simulink model "ChiefMaster_TTC580"  (R2022b)
settings: Solver=FixedStepAuto  StartTime=0.0  StopTime=10  FixedStep=0.01  RelTol=1e-3
values from neighbouring files (symbols this model uses):
  BattBox1_No = single(1)    [Parameters.m]
  BattBox2_No = single(2)    [Parameters.m]
  BattBox3_No = single(3)    [Parameters.m]
  CurrentLB = single(-3)    [Parameters.m]
  CurrentReductionConstant_Lvl0 = single(0.03)    [Parameters.m]
  CurrentReductionConstant_Lvl1 = single(0.05)    [Parameters.m]
  CurrentReductionConstant_Lvl2 = single(0.07)    [Parameters.m]
  CurrentReductionConstant_Lvl3 = single(0.1)    [Parameters.m]
  CurrentUB = single(3)    [Parameters.m]
  DCHV_Minus_In_Delay_ms = single(500)    [Parameters.m]
  FL_sHVC_CellBalanceVoltage_mV = single(3500)    [Parameters.m]
  FL_sInrushCurrent_dividebyzero = single(0.00001)    [Parameters.m]
  FL_u8HMI_BuzzerTimer = uint8(3)    [Parameters.m]
  IP_boActValue = true    [Parameters.m]
  IP_boDeactValue = false    [Parameters.m]
  IP_boInitValue = false    [Parameters.m]
  IP_s_LB = 18000    [Parameters.m]
  IP_s_UB = 22000    [Parameters.m]
  IP_sBatt1_ChargeCurrentMax_Factor = single(0.1)    [Parameters.m]
  IP_sBatt1_ChargeCurrentMax_LB = single(0)    [Parameters.m]
  IP_sBatt1_ChargeCurrentMax_Offset = single(0)    [Parameters.m]
  IP_sBatt1_ChargeCurrentMax_UB = single(6553.5)    [Parameters.m]
  IP_sBatt1_Current_Factor = single(0.1)    [Parameters.m]
  IP_sBatt1_Current_LB = single(-3276.8)    [Parameters.m]
  IP_sBatt1_Current_Offset = single(0)    [Parameters.m]
  IP_sBatt1_Current_UB = single(3276.8)    [Parameters.m]
  IP_sBatt1_DisChargeCurrentMax_Factor = single(0.1)    [Parameters.m]
  IP_sBatt1_DisChargeCurrentMax_LB = single(0)    [Parameters.m]
  IP_sBatt1_DisChargeCurrentMax_Offset = single(0)    [Parameters.m]
  IP_sBatt1_DisChargeCurrentMax_UB = single(6553.5)    [Parameters.m]
  IP_sBatt1_InsulationResistance_Factor = single(5)    [Parameters.m]
  IP_sBatt1_InsulationResistance_LB = single(0)    [Parameters.m]
  IP_sBatt1_InsulationResistance_Offset = single(0)    [Parameters.m]
  IP_sBatt1_InsulationResistance_UB = single(0)    [Parameters.m]
  IP_sBatt1_LiBa_IntResist_mOhm = single(25)    [Parameters.m]
  IP_sBatt1_SOC_Factor = single(1)    [Parameters.m]
  IP_sBatt1_SOC_LB = single(0)    [Parameters.m]
  IP_sBatt1_SOC_Offset = single(0)    [Parameters.m]
  IP_sBatt1_SOC_UB = single(100)    [Parameters.m]
  IP_sBatt1_SOH_Factor = single(1)    [Parameters.m]
  IP_sBatt1_SOH_LB = single(0)    [Parameters.m]
  IP_sBatt1_SOH_Offset = single(0)    [Parameters.m]
  IP_sBatt1_SOH_UB = single(100)    [Parameters.m]
  IP_sBatt1_Ubatt_Factor = single(0.1)    [Parameters.m]
  IP_sBatt1_Ubatt_LB = single(0)    [Parameters.m]
  IP_sBatt1_Ubatt_Offset = single(0)    [Parameters.m]
  IP_sBatt1_Ubatt_UB = single(6553.5)    [Parameters.m]
  IP_sBatt1_UserRi_Factor = single(1)    [Parameters.m]
  IP_sBatt1_UserRi_LB = single(0)    [Parameters.m]
  IP_sBatt1_UserRi_Offset = single(0)    [Parameters.m]
  IP_sBatt1_UserRi_UB = single(255)    [Parameters.m]
  IP_sBatt1_VoltageAtSensor_Factor = single(0.02)    [Parameters.m]
  IP_sBatt1_VoltageAtSensor_LB = single(0)    [Parameters.m]
  IP_sBatt1_VoltageAtSensor_Offset = single(0)    [Parameters.m]
  IP_sBatt1_VoltageAtSensor_UB = single(1310.7)    [Parameters.m]
  IP_sBatt2_LiBa_IntResist_mOhm = single(25)    [Parameters.m]
  IP_sBatt3_LiBa_IntResist_mOhm = single(25)    [Parameters.m]
  IP_sEM_LB = 2000    [Parameters.m]
  IP_sEM_UB = 8000    [Parameters.m]
  IP_sFB_LB = 5000    [Parameters.m]
  IP_sFB_UB = 10000    [Parameters.m]
  IP_sHVIL_LB = 12000    [Parameters.m]
  IP_sHVIL_UB = 15000    [Parameters.m]
  IP_sLoad_Voltage_Factor = single(1)    [Parameters.m]
  IP_sLoad_Voltage_LB = single(0)    [Parameters.m]
  IP_sLoad_Voltage_Offset = single(0)    [Parameters.m]
  IP_sLoad_Voltage_UB = single(65535)    [Parameters.m]
  IP_u8HVIL_Delay_ms = uint8(100)    [Parameters.m]
  IP_u8HW_IN_delay_ms = uint8(100)    [Parameters.m]
  IT_sInsulationSafeValue_kOhm = single(650)    [Parameters.m]
  IT_u8IMD_DelayTime_s = uint8(20)    [Parameters.m]
  MainHV_Minus_In_Delay = single(5)    [Parameters.m]
  MainHV_StatusDelay = single(5)    [Parameters.m]
  NotAvailable_uint16 = single(65535)    [Parameters.m]
  NotAvailable_uint8 = uint8(255)    [Parameters.m]
  OP_boHVIL_Supply = boolean(1)    [Parameters.m]
  SafeCurrentToCloseHV_A = single(5)    [Parameters.m]
  SafeVoltageToCloseHV_V = single(0.5)    [Parameters.m]
  UnexpectedBattChargingFcn_Available = boolean(1)    [Parameters.m]
  Voltage_NA_UB = uint16(65535)    [Parameters.m]
  VoltageSensorAvailableBB1 = boolean(0)    [Parameters.m]
  VoltageSensorAvailableBB2 = boolean(0)    [Parameters.m]
  VoltageSensorAvailableBB3 = boolean(0)    [Parameters.m]
libraries: simulink x184, Library_DataProcessing_v1_1 x167, Library_DataProcessing_v1 x142, libCM x28
(part 11 of 19)

== system ChiefMaster_TTC580/ChiefMaster/Input Processing/LiBa/LiBa_Box1/Subsystem13 ==
  C_LB_Batt1_CellVoltage01_Timeout : Inport
  C_LB_Batt1_CellVoltage02_Timeout : Inport  Port=2
  C_LB_Batt1_CellTemperature_Timeout : Inport  Port=3
  C_LB_Batt1_InsulationMonitor_Timeout : Inport  Port=4
  C_LB_Batt1_Status01_Timeout : Inport  Port=5
  C_LB_Batt1_Status02_Timeout : Inport  Port=6
  C_LB_Batt1_Status03_Timeout : Inport  Port=7
  AND : Logic  Inputs=7  AllPortsSameDT=off  OutDataTypeStr=boolean
  Constant : Constant  OutDataTypeStr=boolean
  Constant1 : Constant  Value=0  OutDataTypeStr=boolean
  NOT{,1..6} (7 alike) : Logic  Operator=NOT  AllPortsSameDT=off  OutDataTypeStr=boolean
  Switch : Switch  Criteria=u2 > Threshold  SaturateOnIntegerOverflow=off  InputSameDT=off
  IP_boLiBa_Batt1_Availability : Outport
  wires:
  NOT6/1 -> AND/7
  NOT5/1 -> AND/6
  C_LB_Batt1_Status03_Timeout/1 -> NOT6/1
  C_LB_Batt1_Status02_Timeout/1 -> NOT5/1
  C_LB_Batt1_Status01_Timeout/1 -> NOT4/1
  Switch/1 -> IP_boLiBa_Batt1_Availability/1  "IP_boLiBa_Batt1_Availability"
  C_LB_Batt1_CellVoltage01_Timeout/1 -> NOT/1
  C_LB_Batt1_CellVoltage02_Timeout/1 -> NOT1/1
  C_LB_Batt1_CellTemperature_Timeout/1 -> NOT2/1
  C_LB_Batt1_InsulationMonitor_Timeout/1 -> NOT3/1
  NOT/1 -> AND/1
  NOT1/1 -> AND/2
  NOT2/1 -> AND/3
  NOT3/1 -> AND/4
  NOT4/1 -> AND/5
  AND/1 -> Switch/2
  Constant/1 -> Switch/1
  Constant1/1 -> Switch/3

== system ChiefMaster_TTC580/ChiefMaster/Input Processing/LiBa/LiBa_Box2/BMS_CellTemperature ==
  C_LB_Batt2_CellTemperature_Msg : Inport
  C_LB_Batt2_CellTemperature_Timeout : Inport  Port=2
  Bus Creator1 : BusCreator  Inputs=7
  Demux : Demux  Outputs=8
  Subsystem : Subsystem
  Subsystem1 : Subsystem
  Subsystem2 : Subsystem
  Subsystem3 : Subsystem
  Subsystem4 : Subsystem
  Subsystem5 : Subsystem
  Subsystem6 : Subsystem
  Terminator1 : Terminator
  IP_LB_Batt2_CellTemperature_DataBus : Outport
  wires:
  Subsystem3/1(IP_LB_BMS_ACT_Cel_T_Min_Cel_DataBus) -> Bus Creator1/4
  [C_LB_BMS_CellTemperature_Timeout] -> Subsystem3/2(C_LB_BMS_CellTemperature_Timeout)
  Demux/4 -> Subsystem3/1(byte3)
  Demux/3 -> Subsystem2/1(byte2)
  Demux/2 -> Subsystem1/1(byte1)
  C_LB_Batt2_CellTemperature_Msg/1 -> Demux/1
  Demux/1 -> Subsystem/1(byte0)
  C_LB_Batt2_CellTemperature_Timeout/1 -> [C_LB_BMS_CellTemperature_Timeout]
  [C_LB_BMS_CellTemperature_Timeout] -> Subsystem/2(C_LB_BMS_CellTemperature_Timeout)
  [C_LB_BMS_CellTemperature_Timeout] -> Subsystem1/2(C_LB_BMS_CellTemperature_Timeout)
  [C_LB_BMS_CellTemperature_Timeout] -> Subsystem2/2(C_LB_BMS_CellTemperature_Timeout)
  Demux/8 -> Terminator1/1
  Subsystem/1(IP_LB_BMS_ACT_Cel_T_Avg_DataBus) -> Bus Creator1/1
  Subsystem1/1(IP_LB_BMS_ACT_Cel_T_Min_Value_DataBus) -> Bus Creator1/2
  Subsystem2/1(IP_LB_BMS_ACT_Cel_T_Max_Value_DataBus) -> Bus Creator1/3
  Bus Creator1/1 -> IP_LB_Batt2_CellTemperature_DataBus/1  "IP_LB_Batt2_CellTemperature_DataBus"
  [C_LB_BMS_CellTemperature_Timeout] -> Subsystem4/2(C_LB_BMS_CellTemperature_Timeout)
  [C_LB_BMS_CellTemperature_Timeout] -> Subsystem5/2(C_LB_BMS_CellTemperature_Timeout)
  [C_LB_BMS_CellTemperature_Timeout] -> Subsystem6/2(C_LB_BMS_CellTemperature_Timeout)
  Demux/5 -> Subsystem4/1(byte1)
  Demux/6 -> Subsystem5/1(byte2)
  Demux/7 -> Subsystem6/1(byte3)
  Subsystem4/1(IP_LB_BMS_ACT_Cel_T_Min_CMU_DataBus) -> Bus Creator1/5
  Subsystem5/1(IP_LB_BMS_ACT_Cel_T_Max_Cel_DataBus) -> Bus Creator1/6
  Subsystem6/1(IP_LB_BMS_ACT_Cel_V_Max_Cel_DataBus) -> Bus Creator1/7

== system ChiefMaster_TTC580/ChiefMaster/Input Processing/LiBa/LiBa_Box2/BMS_CellVoltage01 ==
  C_LB_Batt2_CellVoltage01_Msg : Inport
  C_LB_Batt2_CellVoltage01_Timeout : Inport  Port=2
  Bus Creator1 : BusCreator  Inputs=3
  Demux : Demux  Outputs=8
  Subsystem : Subsystem
  Subsystem1 : Subsystem
  Subsystem2 : Subsystem
  Terminator : Terminator
  Terminator1 : Terminator
  IP_LB_Batt2_CellVoltage01_DataBus : Outport
  wires:
  C_LB_Batt2_CellVoltage01_Msg/1 -> Demux/1
  Demux/1 -> Subsystem/1(byte0)
  Demux/2 -> Subsystem/2(byte1)
  C_LB_Batt2_CellVoltage01_Timeout/1 -> [C_LB_BMS_CellVoltage01_Timeout]
  [C_LB_BMS_CellVoltage01_Timeout] -> Subsystem/3(C_LB_CellVoltage01_Timeout)
  Demux/3 -> Subsystem1/1(byte2)
  Demux/4 -> Subsystem1/2(byte3)
  [C_LB_BMS_CellVoltage01_Timeout] -> Subsystem1/3(C_LB_CellVoltage01_Timeout)
  Demux/5 -> Subsystem2/1(byte4)
  Demux/6 -> Subsystem2/2(byte5)
  [C_LB_BMS_CellVoltage01_Timeout] -> Subsystem2/3(C_LB_CellVoltage01_Timeout)
  Demux/7 -> Terminator/1
  Demux/8 -> Terminator1/1
  Subsystem/1(IP_LB_BMS_ACT_Cel_mV_Min_DataBus) -> Bus Creator1/1
  Subsystem1/1(IP_LB_BMS_ACT_Cel_mV_AVG_DataBus) -> Bus Creator1/2
  Subsystem2/1(IP_LB_BMS_ACT_Cel_mV_Max_DataBus) -> Bus Creator1/3
  Bus Creator1/1 -> IP_LB_Batt2_CellVoltage01_DataBus/1  "IP_LB_Batt2_CellVoltage01_DataBus"

== system ChiefMaster_TTC580/ChiefMaster/Input Processing/LiBa/LiBa_Box2/BMS_CellVoltageNumber ==
  C_LB_Batt2_CellVoltage02_Msg : Inport
  C_LB_Batt2_CellVoltage02_Timeout : Inport  Port=2
  Bus Creator1 : BusCreator  Inputs=4
  Demux : Demux  Outputs=8
  Subsystem : Subsystem
  Subsystem1 : Subsystem
  Subsystem2 : Subsystem
  Subsystem3 : Subsystem
  Terminator{,1..3} (4 alike) : Terminator
  IP_LB_Batt2_CellVoltage02_DataBus : Outport
  wires:
  Bus Creator1/1 -> IP_LB_Batt2_CellVoltage02_DataBus/1  "IP_LB_Batt2_CellVoltage02_DataBus"
  Subsystem2/1(IP_LB_BMS_ACT_Cel_V_Max_Cel_DataBus) -> Bus Creator1/3
  Subsystem1/1(IP_LB_BMS_ACT_Cel_V_Min_CMU_DataBus) -> Bus Creator1/2
  Subsystem/1(IP_LB_BMS_ACT_Cel_V_Min_Cel_DataBus) -> Bus Creator1/1
  Demux/8 -> Terminator1/1
  Demux/7 -> Terminator/1
  [C_LB_BMS_CellVoltage02_Timeout] -> Subsystem2/2(C_LB_CellVoltage02_Timeout)
  [C_LB_BMS_CellVoltage02_Timeout] -> Subsystem1/2(C_LB_CellVoltage02_Timeout)
  [C_LB_BMS_CellVoltage02_Timeout] -> Subsystem/2(C_LB_CellVoltage02_Timeout)
  C_LB_Batt2_CellVoltage02_Timeout/1 -> [C_LB_BMS_CellVoltage02_Timeout]
  Demux/1 -> Subsystem/1(byte0)
  C_LB_Batt2_CellVoltage02_Msg/1 -> Demux/1
  Demux/2 -> Subsystem1/1(byte1)
  Demux/3 -> Subsystem2/1(byte2)
  Demux/4 -> Subsystem3/1(byte3)
  [C_LB_BMS_CellVoltage02_Timeout] -> Subsystem3/2(C_LB_CellVoltage02_Timeout)
  Subsystem3/1(IP_LB_BMS_ACT_Cel_V_Max_CMU_DataBus) -> Bus Creator1/4
  Demux/6 -> Terminator2/1
  Demux/5 -> Terminator3/1

== system ChiefMaster_TTC580/ChiefMaster/Input Processing/LiBa/LiBa_Box2/BMS_InsulationMonitor ==
  C_LB_Batt2_InsulationMonitor_Msg : Inport
  C_LB_Batt2_InsulationMonitor_Timeout : Inport  Port=2
  Bus Creator1 : BusCreator  Inputs=3
  Demux : Demux  Outputs=8
  Subsystem : Subsystem
  Subsystem1 : Subsystem
  Subsystem2 : Subsystem
  Terminator : Terminator
  Terminator1 : Terminator
  IP_LB_Batt2_InsulationMonitor_DataBus : Outport
  wires:
  Bus Creator1/1 -> IP_LB_Batt2_InsulationMonitor_DataBus/1  "IP_LB_Batt2_InsulationMonitor_DataBus"
  Subsystem2/1(IP_LB_BMS_Pack_Leak_Mid_Raw_mV_DataBus) -> Bus Creator1/3
  Subsystem1/1(IP_LB_BMS_Pack_Leak_Neg_Raw_mV_DataBus) -> Bus Creator1/2
  Subsystem/1(IP_LB_BMS_Pack_Leak_Pos_Raw_mV_DataBus) -> Bus Creator1/1
  Demux/8 -> Terminator1/1
  Demux/7 -> Terminator/1
  [C_LB_BMS_InsulationMonitor_Timeout] -> Subsystem2/3(C_LB_BMS_InsulationMonitor_Timeout)
  Demux/6 -> Subsystem2/2(byte5)
  Demux/5 -> Subsystem2/1(byte4)
  [C_LB_BMS_InsulationMonitor_Timeout] -> Subsystem1/3(C_LB_BMS_InsulationMonitor_Timeout)
  Demux/4 -> Subsystem1/2(byte3)
  Demux/3 -> Subsystem1/1(byte2)
  [C_LB_BMS_InsulationMonitor_Timeout] -> Subsystem/3(C_LB_BMS_InsulationMonitor_Timeout)
  C_LB_Batt2_InsulationMonitor_Timeout/1 -> [C_LB_BMS_InsulationMonitor_Timeout]
  Demux/2 -> Subsystem/2(byte1)
  Demux/1 -> Subsystem/1(byte0)
  C_LB_Batt2_InsulationMonitor_Msg/1 -> Demux/1

== system ChiefMaster_TTC580/ChiefMaster/Input Processing/LiBa/LiBa_Box2/BMS_Status01 ==
  C_LB_Batt2_Status01_Msg : Inport
  C_LB_Batt2_Status01_Timeout : Inport  Port=2
  Bus Creator1 : BusCreator  Inputs=9
  Demux : Demux  Outputs=8
  Extract Bits : simulink/Logic and Bit Operations/Extract Bits  bitsToExtract=Range of bits  numBits=8  bitIdxRange=[0 3]  outScalingMode=Preserve fixed-point scaling
  Extract Bits1 : simulink/Logic and Bit Operations/Extract Bits  bitsToExtract=Range of bits  numBits=8  bitIdxRange=[4]  outScalingMode=Preserve fixed-point scaling
  Extract Bits2 : simulink/Logic and Bit Operations/Extract Bits  bitsToExtract=Range of bits  numBits=8  bitIdxRange=[5]  outScalingMode=Preserve fixed-point scaling
  Extract Bits3 : simulink/Logic and Bit Operations/Extract Bits  bitsToExtract=Range of bits  numBits=8  bitIdxRange=[6]  outScalingMode=Preserve fixed-point scaling
  Extract Bits4 : simulink/Logic and Bit Operations/Extract Bits  bitsToExtract=Range of bits  numBits=8  bitIdxRange=[7]  outScalingMode=Preserve fixed-point scaling
  Lib_InputProcessing_dflt0_flag{,1..3} (4 alike) : Library_DataProcessing_v1_1/Lib_InputProcessing_dflt0_flag  SystemSampleTime=-1  VariantActivationTime=update diagram  Latency=0  AutoFrameSizeCalculation=off
  Lib_InputProcessing_state : Library_DataProcessing_v1_1/Lib_InputProcessing_state  SystemSampleTime=-1  VariantActivationTime=update diagram  Latency=0  AutoFrameSizeCalculation=off
  NOT{1..5} (5 alike) : Logic  Operator=NOT  AllPortsSameDT=off  OutDataTypeStr=boolean
  Subsystem1 : Subsystem
  Subsystem2 : Subsystem
  Subsystem3 : Subsystem
  Subsystem4 : Subsystem
  Terminator2 : Terminator
  IP_LB_Batt2_Status01_DataBus : Outport
  wires:
  Bus Creator1/1 -> IP_LB_Batt2_Status01_DataBus/1  "IP_LB_Batt2_Status01_DataBus"
  Subsystem2/1(IP_LB_BMS_IO_State_Output_DataBus) -> Bus Creator1/7
  Subsystem1/1(IP_LB_BMS_IO_state_Input_DataBus) -> Bus Creator1/6
  Lib_InputProcessing_state/1 -> Bus Creator1/1  "IP_u8LB_BMS_Status"
  [C_LB_BMS_Status01_Timeout] -> Subsystem2/2(C_LB_BMS_Status01_Timeout)
  [C_LB_BMS_Status01_Timeout] -> Subsystem1/2(C_LB_BMS_Status01_Timeout)
  [C_LB_BMS_Status01_Timeout] -> NOT1/1
  C_LB_Batt2_Status01_Timeout/1 -> [C_LB_BMS_Status01_Timeout]
  Demux/1 -> Extract Bits4/1, Extract Bits3/1, Extract Bits2/1, Extract Bits1/1, Extract Bits/1
  C_LB_Batt2_Status01_Msg/1 -> Demux/1
  Demux/2 -> Subsystem1/1(byte1)
  Demux/3 -> Subsystem2/1(byte2)
  [C_LB_BMS_Status01_Timeout] -> Subsystem3/3(C_LB_BMS_Status01_Timeout)
  Subsystem3/1(IP_LB_BMS_DYN_Lim_Current_IN_A_DataBus) -> Bus Creator1/8
  Extract Bits/1 -> Lib_InputProcessing_state/1
  Extract Bits1/1 -> Lib_InputProcessing_dflt0_flag/1
  Lib_InputProcessing_dflt0_flag/1 -> Bus Creator1/2  "IP_boLB_BMS_FlagsChargerActive"
  [C_LB_BMS_Status01_Timeout] -> NOT2/1
  [C_LB_BMS_Status01_Timeout] -> NOT3/1
  Extract Bits2/1 -> Lib_InputProcessing_dflt0_flag1/1
  Extract Bits3/1 -> Lib_InputProcessing_dflt0_flag2/1
  [C_LB_BMS_Status01_Timeout] -> NOT4/1
  [C_LB_BMS_Status01_Timeout] -> NOT5/1
  Extract Bits4/1 -> Lib_InputProcessing_dflt0_flag3/1
  Lib_InputProcessing_dflt0_flag1/1 -> Bus Creator1/3  "IP_boLB_BMS_FlagsLoadActive"
  Lib_InputProcessing_dflt0_flag2/1 -> Bus Creator1/4  "IP_boLB_BMS_FlagsPreChargeActive"
  Lib_InputProcessing_dflt0_flag3/1 -> Bus Creator1/5  "IP_boLB_BMS_FlagsBalancingActive"
  Demux/4 -> Terminator2/1
  Demux/5 -> Subsystem3/1(byte4)
  Demux/6 -> Subsystem3/2(byte5)
  Subsystem4/1(IP_LB_BMS_DYN_Lim_Current_OUT_A_DataBus) -> Bus Creator1/9
  Demux/7 -> Subsystem4/1(byte6)
  Demux/8 -> Subsystem4/2(byte7)
  [C_LB_BMS_Status01_Timeout] -> Subsystem4/3(C_LB_BMS_Status01_Timeout)
  NOT1/1 -> Lib_InputProcessing_state/Enable
  NOT2/1 -> Lib_InputProcessing_dflt0_flag/Enable
  NOT3/1 -> Lib_InputProcessing_dflt0_flag1/Enable
  NOT4/1 -> Lib_InputProcessing_dflt0_flag2/Enable
  NOT5/1 -> Lib_InputProcessing_dflt0_flag3/Enable

== system ChiefMaster_TTC580/ChiefMaster/Input Processing/LiBa/LiBa_Box2/BMS_Status02 ==
  C_LB_Batt2_Status02_Msg : Inport
  C_LB_Batt2_Status02_Timeout : Inport  Port=2
  Bus Creator1 : BusCreator  Inputs=3
  Demux : Demux  Outputs=8
  Subsystem1 : Subsystem
  Subsystem2 : Subsystem
  Subsystem3 : Subsystem
  IP_LB_Batt2_Status02_DataBus : Outport
  wires:
  [C_LB_BMS_Status02_Timeout] -> Subsystem3/3(C_LB_BMS_Status02_Timeout)
  C_LB_Batt2_Status02_Msg/1 -> Demux/1
  C_LB_Batt2_Status02_Timeout/1 -> [C_LB_BMS_Status02_Timeout]
  Bus Creator1/1 -> IP_LB_Batt2_Status02_DataBus/1  "IP_LB_Batt2_Status02_DataBus"
  Demux/1 -> Subsystem3/1(byte0)
  Demux/2 -> Subsystem3/2(byte1)
  Subsystem3/1(IP_LB_BMS_Pack_Q_SOC_Internal_DataBus) -> Bus Creator1/1
  Demux/3 -> Subsystem1/1(byte2)
  Demux/5 -> Subsystem1/3(byte4)
  Demux/6 -> Subsystem1/4(byte5)
  [C_LB_BMS_Status02_Timeout] -> Subsystem1/5(C_LB_BMS_Status02_Timeout)
  Demux/4 -> Subsystem1/2(byte3)
  Subsystem1/1(IP_LB_BMS_Pack_Current_Master_mA_DataBus) -> Bus Creator1/2
  [C_LB_BMS_Status02_Timeout] -> Subsystem2/3(C_LB_BMS_Status02_Timeout)
  Demux/8 -> Subsystem2/2(byte7)
  Demux/7 -> Subsystem2/1(byte6)
  Subsystem2/1(IP_LB_BMS_Pack_V_Cells_DataBus) -> Bus Creator1/3

== system ChiefMaster_TTC580/ChiefMaster/Input Processing/LiBa/LiBa_Box2/BMS_Status03 ==
  C_LB_Batt2_Status03_Msg : Inport
  C_LB_Batt2_Status03_Timeout : Inport  Port=2
  Bus Creator1 : BusCreator  Inputs=1
  Demux : Demux  Outputs=8
  Subsystem3 : Subsystem
  Terminator{,1..5} (6 alike) : Terminator
  IP_LB_Batt2_Status03_DataBus : Outport
  wires:
  Subsystem3/1(IP_LB_BMS_REQ_Charger_Current_A_DataBus) -> Bus Creator1/1
  Demux/2 -> Subsystem3/2(byte1)
  Demux/1 -> Subsystem3/1(byte0)
  Bus Creator1/1 -> IP_LB_Batt2_Status03_DataBus/1  "IP_LB_Batt2_Status03_DataBus"
  C_LB_Batt2_Status03_Timeout/1 -> [C_LB_BMS_Status03_Timeout]
  C_LB_Batt2_Status03_Msg/1 -> Demux/1
  [C_LB_BMS_Status03_Timeout] -> Subsystem3/3(C_LB_BMS_Status03_Timeout)
  Demux/3 -> Terminator/1
  Demux/4 -> Terminator1/1
  Demux/5 -> Terminator2/1
  Demux/6 -> Terminator3/1
  Demux/7 -> Terminator4/1
  Demux/8 -> Terminator5/1

== system ChiefMaster_TTC580/ChiefMaster/Input Processing/LiBa/LiBa_Box2/Subsystem13 ==
  C_LB_Batt1_CellVoltage01_Timeout : Inport
  C_LB_Batt1_CellVoltage02_Timeout : Inport  Port=2
  C_LB_Batt1_CellTemperature_Timeout : Inport  Port=3
  C_LB_Batt1_InsulationMonitor_Timeout : Inport  Port=4
  C_LB_Batt1_Status01_Timeout : Inport  Port=5
  C_LB_Batt1_Status02_Timeout : Inport  Port=6
  C_LB_Batt1_Status03_Timeout : Inport  Port=7
  AND : Logic  Inputs=7  AllPortsSameDT=off  OutDataTypeStr=boolean
  Constant : Constant  OutDataTypeStr=boolean
  Constant1 : Constant  Value=0  OutDataTypeStr=boolean
  NOT{,1..6} (7 alike) : Logic  Operator=NOT  AllPortsSameDT=off  OutDataTypeStr=boolean
  Switch : Switch  Criteria=u2 > Threshold  SaturateOnIntegerOverflow=off  InputSameDT=off
  IP_boLiBa_Batt2_Availability : Outport
  wires:
  AND/1 -> Switch/2
  NOT6/1 -> AND/7
  NOT5/1 -> AND/6
  C_LB_Batt1_Status03_Timeout/1 -> NOT6/1
  C_LB_Batt1_Status02_Timeout/1 -> NOT5/1
  C_LB_Batt1_Status01_Timeout/1 -> NOT4/1
  Switch/1 -> IP_boLiBa_Batt2_Availability/1  "IP_boLiBa_Batt2_Availability"
  C_LB_Batt1_CellVoltage01_Timeout/1 -> NOT/1
  C_LB_Batt1_CellVoltage02_Timeout/1 -> NOT1/1
  C_LB_Batt1_CellTemperature_Timeout/1 -> NOT2/1
  C_LB_Batt1_InsulationMonitor_Timeout/1 -> NOT3/1
  NOT/1 -> AND/1
  NOT1/1 -> AND/2
  NOT2/1 -> AND/3
  NOT3/1 -> AND/4
  NOT4/1 -> AND/5
  Constant/1 -> Switch/1
  Constant1/1 -> Switch/3

== system ChiefMaster_TTC580/ChiefMaster/Input Processing/LiBa/LiBa_Box3/BMS_CellTemperature ==
  C_LB_Batt3_CellTemperature_Msg : Inport
  C_LB_Batt3_CellTemperature_Timeout : Inport  Port=2
  Bus Creator1 : BusCreator  Inputs=7
  Demux : Demux  Outputs=8
  Subsystem : Subsystem
  Subsystem1 : Subsystem
  Subsystem2 : Subsystem
  Subsystem3 : Subsystem
  Subsystem4 : Subsystem
  Subsystem5 : Subsystem
  Subsystem6 : Subsystem
  Terminator1 : Terminator
  IP_LB_Batt3_CellTemperature_DataBus : Outport
  wires:
  Subsystem3/1(IP_LB_BMS_ACT_Cel_T_Min_Cel_DataBus) -> Bus Creator1/4
  [C_LB_BMS_CellTemperature_Timeout] -> Subsystem3/2(C_LB_BMS_CellTemperature_Timeout)
  Demux/4 -> Subsystem3/1(byte3)
  Demux/3 -> Subsystem2/1(byte2)
  Demux/2 -> Subsystem1/1(byte1)
  C_LB_Batt3_CellTemperature_Msg/1 -> Demux/1
  Demux/1 -> Subsystem/1(byte0)
  C_LB_Batt3_CellTemperature_Timeout/1 -> [C_LB_BMS_CellTemperature_Timeout]
  [C_LB_BMS_CellTemperature_Timeout] -> Subsystem/2(C_LB_BMS_CellTemperature_Timeout)
  [C_LB_BMS_CellTemperature_Timeout] -> Subsystem1/2(C_LB_BMS_CellTemperature_Timeout)
  [C_LB_BMS_CellTemperature_Timeout] -> Subsystem2/2(C_LB_BMS_CellTemperature_Timeout)
  Demux/8 -> Terminator1/1
  Subsystem/1(IP_LB_BMS_ACT_Cel_T_Avg_DataBus) -> Bus Creator1/1
  Subsystem1/1(IP_LB_BMS_ACT_Cel_T_Min_Value_DataBus) -> Bus Creator1/2
  Subsystem2/1(IP_LB_BMS_ACT_Cel_T_Max_Value_DataBus) -> Bus Creator1/3
  Bus Creator1/1 -> IP_LB_Batt3_CellTemperature_DataBus/1  "IP_LB_Batt3_CellTemperature_DataBus"
  [C_LB_BMS_CellTemperature_Timeout] -> Subsystem4/2(C_LB_BMS_CellTemperature_Timeout)
  [C_LB_BMS_CellTemperature_Timeout] -> Subsystem5/2(C_LB_BMS_CellTemperature_Timeout)
  [C_LB_BMS_CellTemperature_Timeout] -> Subsystem6/2(C_LB_BMS_CellTemperature_Timeout)
  Demux/5 -> Subsystem4/1(byte1)
  Demux/6 -> Subsystem5/1(byte2)
  Demux/7 -> Subsystem6/1(byte3)
  Subsystem4/1(IP_LB_BMS_ACT_Cel_T_Min_CMU_DataBus) -> Bus Creator1/5
  Subsystem5/1(IP_LB_BMS_ACT_Cel_T_Max_Cel_DataBus) -> Bus Creator1/6
  Subsystem6/1(IP_LB_BMS_ACT_Cel_V_Max_Cel_DataBus) -> Bus Creator1/7

== system ChiefMaster_TTC580/ChiefMaster/Input Processing/LiBa/LiBa_Box3/BMS_CellVoltage01 ==
  C_LB_Batt3_CellVoltage01_Msg : Inport
  C_LB_Batt3_CellVoltage01_Timeout : Inport  Port=2
  Bus Creator1 : BusCreator  Inputs=3
  Demux : Demux  Outputs=8
  Subsystem : Subsystem
  Subsystem1 : Subsystem
  Subsystem2 : Subsystem
  Terminator : Terminator
  Terminator1 : Terminator
  IP_LB_Batt3_CellVoltage01_DataBus : Outport
  wires:
  C_LB_Batt3_CellVoltage01_Msg/1 -> Demux/1
  Demux/1 -> Subsystem/1(byte0)
  Demux/2 -> Subsystem/2(byte1)
  C_LB_Batt3_CellVoltage01_Timeout/1 -> [C_LB_BMS_CellVoltage01_Timeout]
  [C_LB_BMS_CellVoltage01_Timeout] -> Subsystem/3(C_LB_CellVoltage01_Timeout)
  Demux/3 -> Subsystem1/1(byte2)
  Demux/4 -> Subsystem1/2(byte3)
  [C_LB_BMS_CellVoltage01_Timeout] -> Subsystem1/3(C_LB_CellVoltage01_Timeout)
  Demux/5 -> Subsystem2/1(byte4)
  Demux/6 -> Subsystem2/2(byte5)
  [C_LB_BMS_CellVoltage01_Timeout] -> Subsystem2/3(C_LB_CellVoltage01_Timeout)
  Demux/7 -> Terminator/1
  Demux/8 -> Terminator1/1
  Subsystem/1(IP_LB_BMS_ACT_Cel_mV_Min_DataBus) -> Bus Creator1/1
  Subsystem1/1(IP_LB_BMS_ACT_Cel_mV_AVG_DataBus) -> Bus Creator1/2
  Subsystem2/1(IP_LB_BMS_ACT_Cel_mV_Max_DataBus) -> Bus Creator1/3
  Bus Creator1/1 -> IP_LB_Batt3_CellVoltage01_DataBus/1  "IP_LB_Batt3_CellVoltage01_DataBus"

== system ChiefMaster_TTC580/ChiefMaster/Input Processing/LiBa/LiBa_Box3/BMS_CellVoltageNumber ==
  C_LB_Batt3_CellVoltage02_Msg : Inport
  C_LB_Batt3_CellVoltage02_Timeout : Inport  Port=2
  Bus Creator1 : BusCreator  Inputs=4
  Demux : Demux  Outputs=8
  Subsystem : Subsystem
  Subsystem1 : Subsystem
  Subsystem2 : Subsystem
  Subsystem3 : Subsystem
  Terminator{,1..3} (4 alike) : Terminator
  IP_LB_Batt3_CellVoltage02_DataBus : Outport
  wires:
  Bus Creator1/1 -> IP_LB_Batt3_CellVoltage02_DataBus/1  "IP_LB_Batt3_CellVoltage02_DataBus"
  Subsystem2/1(IP_LB_BMS_ACT_Cel_V_Max_Cel_DataBus) -> Bus Creator1/3
  Subsystem1/1(IP_LB_BMS_ACT_Cel_V_Min_CMU_DataBus) -> Bus Creator1/2
  Subsystem/1(IP_LB_BMS_ACT_Cel_V_Min_Cel_DataBus) -> Bus Creator1/1
  Demux/8 -> Terminator1/1
  Demux/7 -> Terminator/1
  [C_LB_BMS_CellVoltage02_Timeout] -> Subsystem2/2(C_LB_CellVoltage02_Timeout)
  [C_LB_BMS_CellVoltage02_Timeout] -> Subsystem1/2(C_LB_CellVoltage02_Timeout)
  [C_LB_BMS_CellVoltage02_Timeout] -> Subsystem/2(C_LB_CellVoltage02_Timeout)
  C_LB_Batt3_CellVoltage02_Timeout/1 -> [C_LB_BMS_CellVoltage02_Timeout]
  Demux/1 -> Subsystem/1(byte0)
  C_LB_Batt3_CellVoltage02_Msg/1 -> Demux/1
  Demux/2 -> Subsystem1/1(byte1)
  Demux/3 -> Subsystem2/1(byte2)
  Demux/4 -> Subsystem3/1(byte3)
  [C_LB_BMS_CellVoltage02_Timeout] -> Subsystem3/2(C_LB_CellVoltage02_Timeout)
  Subsystem3/1(IP_LB_BMS_ACT_Cel_V_Max_CMU_DataBus) -> Bus Creator1/4
  Demux/6 -> Terminator2/1
  Demux/5 -> Terminator3/1

== system ChiefMaster_TTC580/ChiefMaster/Input Processing/LiBa/LiBa_Box3/BMS_InsulationMonitor ==
  C_LB_Batt3_InsulationMonitor_Msg : Inport
  C_LB_Batt3_InsulationMonitor_Timeout : Inport  Port=2
  Bus Creator1 : BusCreator  Inputs=3
  Demux : Demux  Outputs=8
  Subsystem : Subsystem
  Subsystem1 : Subsystem
  Subsystem2 : Subsystem
  Terminator : Terminator
  Terminator1 : Terminator
  IP_LB_Batt3_InsulationMonitor_DataBus : Outport
  wires:
  Bus Creator1/1 -> IP_LB_Batt3_InsulationMonitor_DataBus/1  "IP_LB_Batt3_InsulationMonitor_DataBus"
  Subsystem2/1(IP_LB_BMS_Pack_Leak_Mid_Raw_mV_DataBus) -> Bus Creator1/3
  Subsystem1/1(IP_LB_BMS_Pack_Leak_Neg_Raw_mV_DataBus) -> Bus Creator1/2
  Subsystem/1(IP_LB_BMS_Pack_Leak_Pos_Raw_mV_DataBus) -> Bus Creator1/1
  Demux/8 -> Terminator1/1
  Demux/7 -> Terminator/1
  [C_LB_BMS_InsulationMonitor_Timeout] -> Subsystem2/3(C_LB_BMS_InsulationMonitor_Timeout)
  Demux/6 -> Subsystem2/2(byte5)
  Demux/5 -> Subsystem2/1(byte4)
  [C_LB_BMS_InsulationMonitor_Timeout] -> Subsystem1/3(C_LB_BMS_InsulationMonitor_Timeout)
  Demux/4 -> Subsystem1/2(byte3)
  Demux/3 -> Subsystem1/1(byte2)
  [C_LB_BMS_InsulationMonitor_Timeout] -> Subsystem/3(C_LB_BMS_InsulationMonitor_Timeout)
  C_LB_Batt3_InsulationMonitor_Timeout/1 -> [C_LB_BMS_InsulationMonitor_Timeout]
  Demux/2 -> Subsystem/2(byte1)
  Demux/1 -> Subsystem/1(byte0)
  C_LB_Batt3_InsulationMonitor_Msg/1 -> Demux/1

== system ChiefMaster_TTC580/ChiefMaster/Input Processing/LiBa/LiBa_Box3/BMS_Status01 ==
  C_LB_Batt3_Status01_Msg : Inport
  C_LB_Batt3_Status01_Timeout : Inport  Port=2
  Bus Creator1 : BusCreator  Inputs=9
  Demux : Demux  Outputs=8
  Extract Bits : simulink/Logic and Bit Operations/Extract Bits  bitsToExtract=Range of bits  numBits=8  bitIdxRange=[0 3]  outScalingMode=Preserve fixed-point scaling
  Extract Bits1 : simulink/Logic and Bit Operations/Extract Bits  bitsToExtract=Range of bits  numBits=8  bitIdxRange=[4]  outScalingMode=Preserve fixed-point scaling
  Extract Bits2 : simulink/Logic and Bit Operations/Extract Bits  bitsToExtract=Range of bits  numBits=8  bitIdxRange=[5]  outScalingMode=Preserve fixed-point scaling
  Extract Bits3 : simulink/Logic and Bit Operations/Extract Bits  bitsToExtract=Range of bits  numBits=8  bitIdxRange=[6]  outScalingMode=Preserve fixed-point scaling
  Extract Bits4 : simulink/Logic and Bit Operations/Extract Bits  bitsToExtract=Range of bits  numBits=8  bitIdxRange=[7]  outScalingMode=Preserve fixed-point scaling
  Lib_InputProcessing_dflt0_flag{,1..3} (4 alike) : Library_DataProcessing_v1_1/Lib_InputProcessing_dflt0_flag  SystemSampleTime=-1  VariantActivationTime=update diagram  Latency=0  AutoFrameSizeCalculation=off
  Lib_InputProcessing_state : Library_DataProcessing_v1_1/Lib_InputProcessing_state  SystemSampleTime=-1  VariantActivationTime=update diagram  Latency=0  AutoFrameSizeCalculation=off
  NOT{1..5} (5 alike) : Logic  Operator=NOT  AllPortsSameDT=off  OutDataTypeStr=boolean
  Subsystem1 : Subsystem
  Subsystem2 : Subsystem
  Subsystem3 : Subsystem
  Subsystem4 : Subsystem
  Terminator2 : Terminator
  IP_LB_Batt3_Status01_DataBus : Outport
  wires:
  Bus Creator1/1 -> IP_LB_Batt3_Status01_DataBus/1  "IP_LB_Batt3_Status01_DataBus"
  Subsystem2/1(IP_LB_BMS_IO_State_Output_DataBus) -> Bus Creator1/7
  Subsystem1/1(IP_LB_BMS_IO_state_Input_DataBus) -> Bus Creator1/6
  Lib_InputProcessing_state/1 -> Bus Creator1/1  "IP_u8LB_BMS_Status"
  [C_LB_BMS_Status01_Timeout] -> Subsystem2/2(C_LB_BMS_Status01_Timeout)
  [C_LB_BMS_Status01_Timeout] -> Subsystem1/2(C_LB_BMS_Status01_Timeout)
  [C_LB_BMS_Status01_Timeout] -> NOT1/1
  C_LB_Batt3_Status01_Timeout/1 -> [C_LB_BMS_Status01_Timeout]
  Demux/1 -> Extract Bits4/1, Extract Bits3/1, Extract Bits2/1, Extract Bits1/1, Extract Bits/1
  C_LB_Batt3_Status01_Msg/1 -> Demux/1
  Demux/2 -> Subsystem1/1(byte1)
  Demux/3 -> Subsystem2/1(byte2)
  [C_LB_BMS_Status01_Timeout] -> Subsystem3/3(C_LB_BMS_Status01_Timeout)
  Subsystem3/1(IP_LB_BMS_DYN_Lim_Current_IN_A_DataBus) -> Bus Creator1/8
  Extract Bits/1 -> Lib_InputProcessing_state/1
  Extract Bits1/1 -> Lib_InputProcessing_dflt0_flag/1
  Lib_InputProcessing_dflt0_flag/1 -> Bus Creator1/2  "IP_boLB_BMS_FlagsChargerActive"
  [C_LB_BMS_Status01_Timeout] -> NOT2/1
  [C_LB_BMS_Status01_Timeout] -> NOT3/1
  Extract Bits2/1 -> Lib_InputProcessing_dflt0_flag1/1
  Extract Bits3/1 -> Lib_InputProcessing_dflt0_flag2/1
  [C_LB_BMS_Status01_Timeout] -> NOT4/1
  [C_LB_BMS_Status01_Timeout] -> NOT5/1
  Extract Bits4/1 -> Lib_InputProcessing_dflt0_flag3/1
  Lib_InputProcessing_dflt0_flag1/1 -> Bus Creator1/3  "IP_boLB_BMS_FlagsLoadActive"
  Lib_InputProcessing_dflt0_flag2/1 -> Bus Creator1/4  "IP_boLB_BMS_FlagsPreChargeActive"
  Lib_InputProcessing_dflt0_flag3/1 -> Bus Creator1/5  "IP_boLB_BMS_FlagsBalancingActive"
  Demux/4 -> Terminator2/1
  Demux/5 -> Subsystem3/1(byte4)
  Demux/6 -> Subsystem3/2(byte5)
  Subsystem4/1(IP_LB_BMS_DYN_Lim_Current_OUT_A_DataBus) -> Bus Creator1/9
  Demux/7 -> Subsystem4/1(byte6)
  Demux/8 -> Subsystem4/2(byte7)
  [C_LB_BMS_Status01_Timeout] -> Subsystem4/3(C_LB_BMS_Status01_Timeout)
  NOT1/1 -> Lib_InputProcessing_state/Enable
  NOT2/1 -> Lib_InputProcessing_dflt0_flag/Enable
  NOT3/1 -> Lib_InputProcessing_dflt0_flag1/Enable
  NOT4/1 -> Lib_InputProcessing_dflt0_flag2/Enable
  NOT5/1 -> Lib_InputProcessing_dflt0_flag3/Enable

== system ChiefMaster_TTC580/ChiefMaster/Input Processing/LiBa/LiBa_Box3/BMS_Status02 ==
  C_LB_Batt3_Status02_Msg : Inport
  C_LB_Batt3_Status02_Timeout : Inport  Port=2
  Bus Creator1 : BusCreator  Inputs=3
  Demux : Demux  Outputs=8
  Subsystem1 : Subsystem
  Subsystem2 : Subsystem
  Subsystem3 : Subsystem
  IP_LB_Batt3_Status02_DataBus : Outport
  wires:
  [C_LB_BMS_Status02_Timeout] -> Subsystem3/3(C_LB_BMS_Status02_Timeout)
  C_LB_Batt3_Status02_Msg/1 -> Demux/1
  C_LB_Batt3_Status02_Timeout/1 -> [C_LB_BMS_Status02_Timeout]
  Bus Creator1/1 -> IP_LB_Batt3_Status02_DataBus/1  "IP_LB_Batt3_Status02_DataBus"
  Demux/1 -> Subsystem3/1(byte0)
  Demux/2 -> Subsystem3/2(byte1)
  Subsystem3/1(IP_LB_BMS_Pack_Q_SOC_Internal_DataBus) -> Bus Creator1/1
  Demux/3 -> Subsystem1/1(byte2)
  Demux/5 -> Subsystem1/3(byte4)
  Demux/6 -> Subsystem1/4(byte5)
  [C_LB_BMS_Status02_Timeout] -> Subsystem1/5(C_LB_BMS_Status02_Timeout)
  Demux/4 -> Subsystem1/2(byte3)
  Subsystem1/1(IP_LB_BMS_Pack_Current_Master_mA_DataBus) -> Bus Creator1/2
  [C_LB_BMS_Status02_Timeout] -> Subsystem2/3(C_LB_BMS_Status02_Timeout)
  Demux/8 -> Subsystem2/2(byte7)
  Demux/7 -> Subsystem2/1(byte6)
  Subsystem2/1(IP_LB_BMS_Pack_V_Cells_DataBus) -> Bus Creator1/3

== system ChiefMaster_TTC580/ChiefMaster/Input Processing/LiBa/LiBa_Box3/BMS_Status03 ==
  C_LB_Batt3_Status03_Msg : Inport
  C_LB_Batt3_Status03_Timeout : Inport  Port=2
  Bus Creator1 : BusCreator  Inputs=1
  Demux : Demux  Outputs=8
  Subsystem3 : Subsystem
  Terminator{,1..5} (6 alike) : Terminator
  "IP_LB_Batt3_Status03_DataBus " : Outport
  wires:
  Subsystem3/1(IP_LB_BMS_REQ_Charger_Current_A_DataBus) -> Bus Creator1/1
  Demux/2 -> Subsystem3/2(byte1)
  Demux/1 -> Subsystem3/1(byte0)
  Bus Creator1/1 -> "IP_LB_Batt3_Status03_DataBus "/1  "IP_LB_Batt3_Status03_DataBus"
  C_LB_Batt3_Status03_Timeout/1 -> [C_LB_BMS_Status03_Timeout]
  C_LB_Batt3_Status03_Msg/1 -> Demux/1
  [C_LB_BMS_Status03_Timeout] -> Subsystem3/3(C_LB_BMS_Status03_Timeout)
  Demux/3 -> Terminator/1
  Demux/4 -> Terminator1/1
  Demux/5 -> Terminator2/1
  Demux/6 -> Terminator3/1
  Demux/7 -> Terminator4/1
  Demux/8 -> Terminator5/1

== system ChiefMaster_TTC580/ChiefMaster/Input Processing/LiBa/LiBa_Box3/Subsystem13 ==
  C_LB_Batt1_CellVoltage01_Timeout : Inport
  C_LB_Batt1_CellVoltage02_Timeout : Inport  Port=2
  C_LB_Batt1_CellTemperature_Timeout : Inport  Port=3
  C_LB_Batt1_InsulationMonitor_Timeout : Inport  Port=4
  C_LB_Batt1_Status01_Timeout : Inport  Port=5
  C_LB_Batt1_Status02_Timeout : Inport  Port=6
  C_LB_Batt1_Status03_Timeout : Inport  Port=7
  AND : Logic  Inputs=7  AllPortsSameDT=off  OutDataTypeStr=boolean
  Constant : Constant  OutDataTypeStr=boolean
  Constant1 : Constant  Value=0  OutDataTypeStr=boolean
  NOT{,1..6} (7 alike) : Logic  Operator=NOT  AllPortsSameDT=off  OutDataTypeStr=boolean
  Switch : Switch  Criteria=u2 > Threshold  SaturateOnIntegerOverflow=off  InputSameDT=off
  IP_boLiBa_Batt3_Availability : Outport
  wires:
  AND/1 -> Switch/2
  Constant1/1 -> Switch/3
  Constant/1 -> Switch/1
  NOT6/1 -> AND/7
  NOT5/1 -> AND/6
  C_LB_Batt1_Status03_Timeout/1 -> NOT6/1
  C_LB_Batt1_Status02_Timeout/1 -> NOT5/1
  C_LB_Batt1_Status01_Timeout/1 -> NOT4/1
  Switch/1 -> IP_boLiBa_Batt3_Availability/1  "IP_boLiBa_Batt3_Availability"
  C_LB_Batt1_CellVoltage01_Timeout/1 -> NOT/1
  C_LB_Batt1_CellVoltage02_Timeout/1 -> NOT1/1
  C_LB_Batt1_CellTemperature_Timeout/1 -> NOT2/1
  C_LB_Batt1_InsulationMonitor_Timeout/1 -> NOT3/1
  NOT/1 -> AND/1
  NOT1/1 -> AND/2
  NOT2/1 -> AND/3
  NOT3/1 -> AND/4
  NOT4/1 -> AND/5

== system ChiefMaster_TTC580/ChiefMaster/Input Translation/Battery Signals/BatteryPackSignals/Subsystem ==
  IP_boBMS_SDError_BB1 : Inport
  Signal Copy : SignalConversion  OverrideOpt=off
  IT_boBMS_SDError_BB1 : Outport
  wires:
  Signal Copy/1 -> IT_boBMS_SDError_BB1/1  "IT_boBMS_SDError_BB1"
  IP_boBMS_SDError_BB1/1 -> Signal Copy/1

== system ChiefMaster_TTC580/ChiefMaster/Input Translation/Battery Signals/BatteryPackSignals/Subsystem1 ==
  IP_boBMS_SDError_BB2 : Inport
  Signal Copy : SignalConversion  OverrideOpt=off
  IT_boBMS_SDError_BB2 : Outport
  wires:
  IP_boBMS_SDError_BB2/1 -> Signal Copy/1
  Signal Copy/1 -> IT_boBMS_SDError_BB2/1  "IT_boBMS_SDError_BB2"

== system ChiefMaster_TTC580/ChiefMaster/Input Translation/Battery Signals/BatteryPackSignals/Subsystem2 ==
  IP_boBMS_SDError_BB3 : Inport
  Signal Copy : SignalConversion  OverrideOpt=off
  IT_boBMS_SDError_BB3 : Outport
  wires:
  Signal Copy/1 -> IT_boBMS_SDError_BB3/1  "IT_boBMS_SDError_BB3"
  IP_boBMS_SDError_BB3/1 -> Signal Copy/1

== system ChiefMaster_TTC580/ChiefMaster/Input Translation/Battery Signals/BatteryPackSignals/Subsystem3 ==
  IP_boBMS_Batt1_Availability : Inport
  IP_boBMS_Batt2_Availability : Inport  Port=2
  IP_boBMS_Batt3_Availability : Inport  Port=3
  IT_boSig_SDError_BB1 : Inport  Port=4
  IT_boSig_SDError_BB2 : Inport  Port=5
  IT_boSig_SDError_BB3 : Inport  Port=6
  AND : Logic  AllPortsSameDT=off  OutDataTypeStr=boolean
  AND1 : Logic  AllPortsSameDT=off  OutDataTypeStr=boolean
  AND2 : Logic  AllPortsSameDT=off  OutDataTypeStr=boolean
  Add : Sum  Inputs=+++
  NOT : Logic  Operator=NOT  AllPortsSameDT=off  OutDataTypeStr=boolean
  NOT1 : Logic  Operator=NOT  AllPortsSameDT=off  OutDataTypeStr=boolean
  NOT2 : Logic  Operator=NOT  AllPortsSameDT=off  OutDataTypeStr=boolean
  IT_u8BMS_No_of_Battery_Usable : Outport
  wires:
  NOT1/1 -> AND1/2
  IP_boBMS_Batt2_Availability/1 -> AND1/1
  NOT/1 -> AND/2
  AND1/1 -> Add/2
  AND2/1 -> Add/3
  NOT2/1 -> AND2/2
  AND/1 -> Add/1
  IT_boSig_SDError_BB2/1 -> NOT1/1
  IT_boSig_SDError_BB3/1 -> NOT2/1
  Add/1 -> IT_u8BMS_No_of_Battery_Usable/1  "IT_u8BMS_No_of_Battery_Usable"
  IT_boSig_SDError_BB1/1 -> NOT/1
  IP_boBMS_Batt3_Availability/1 -> AND2/1
  IP_boBMS_Batt1_Availability/1 -> AND/1

== system ChiefMaster_TTC580/ChiefMaster/Input Translation/Battery Signals/BatteryPackSignals/Subsystem4 ==
  IP_boBMS_InsulationResistance_OK : Inport
  IP_boBMS_Batt1_Availability : Inport  Port=2
  AND : Logic  AllPortsSameDT=off  OutDataTypeStr=boolean
  IMDOK_Input_Delay : Stateflow chart  TreatAsAtomicUnit=on
  NOT : Logic  Operator=NOT  AllPortsSameDT=off  OutDataTypeStr=boolean
  IP_boBMS_InsulationSDError_B1 : Outport
  wires:
  IP_boBMS_InsulationResistance_OK/1 -> NOT/1
  IP_boBMS_Batt1_Availability/1 -> AND/2
  AND/1 -> IP_boBMS_InsulationSDError_B1/1
  NOT/1 -> IMDOK_Input_Delay/1(In)
  IMDOK_Input_Delay/1(out) -> AND/1

== system ChiefMaster_TTC580/ChiefMaster/Input Translation/Battery Signals/BatteryPackSignals/Subsystem5 ==
  IP_boBMS_InsulationResistance_OK : Inport
  IP_boBMS_Batt2_Availability : Inport  Port=2
  AND : Logic  AllPortsSameDT=off  OutDataTypeStr=boolean
  IMDOK_Input_Delay : Stateflow chart  TreatAsAtomicUnit=on
  NOT : Logic  Operator=NOT  AllPortsSameDT=off  OutDataTypeStr=boolean
  IP_boBMS_InsulationSDError_B2 : Outport
  wires:
  NOT/1 -> IMDOK_Input_Delay/1(In)
  AND/1 -> IP_boBMS_InsulationSDError_B2/1
  IP_boBMS_Batt2_Availability/1 -> AND/2
  IP_boBMS_InsulationResistance_OK/1 -> NOT/1
  IMDOK_Input_Delay/1(out) -> AND/1

== system ChiefMaster_TTC580/ChiefMaster/Input Translation/Battery Signals/BatteryPackSignals/Subsystem6 ==
  IP_boBMS_InsulationResistance_OK : Inport
  IP_boBMS_Batt3_Availability : Inport  Port=2
  AND : Logic  AllPortsSameDT=off  OutDataTypeStr=boolean
  IMDOK_Input_Delay : Stateflow chart  TreatAsAtomicUnit=on
  NOT : Logic  Operator=NOT  AllPortsSameDT=off  OutDataTypeStr=boolean
  IP_boBMS_InsulationSDError_B3 : Outport
  wires:
  IP_boBMS_InsulationResistance_OK/1 -> NOT/1
  IP_boBMS_Batt3_Availability/1 -> AND/2
  AND/1 -> IP_boBMS_InsulationSDError_B3/1
  NOT/1 -> IMDOK_Input_Delay/1(In)
  IMDOK_Input_Delay/1(out) -> AND/1

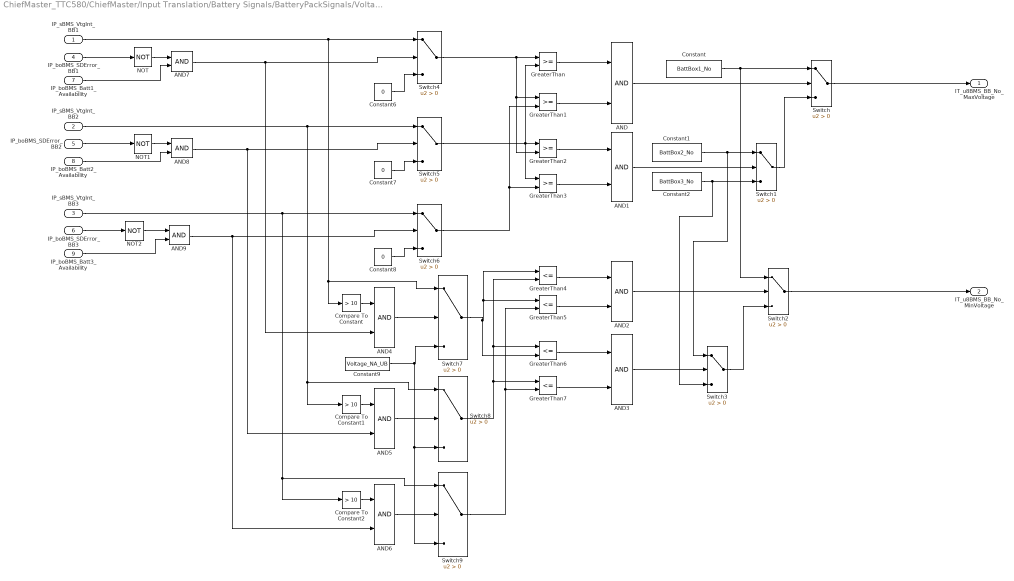
== system ChiefMaster_TTC580/ChiefMaster/Input Translation/Battery Signals/BatteryPackSignals/VoltageDetermination ==
  IP_sBMS_VtgInt_BB1 : Inport
  IP_sBMS_VtgInt_BB2 : Inport  Port=2
  IP_sBMS_VtgInt_BB3 : Inport  Port=3
  IP_boBMS_SDError_BB1 : Inport  Port=4
  IP_boBMS_SDError_BB2 : Inport  Port=5
  IP_boBMS_SDError_BB3 : Inport  Port=6
  IP_boBMS_Batt1_Availability : Inport  Port=7
  IP_boBMS_Batt2_Availability : Inport  Port=8
  IP_boBMS_Batt3_Availability : Inport  Port=9
  AND{,1..9} (10 alike) : Logic  AllPortsSameDT=off  OutDataTypeStr=boolean
  Compare To Constant : simulink/Logic and Bit Operations/Compare To Constant  relop=>  const=10  OutDataTypeStr=boolean
  Compare To Constant1 : simulink/Logic and Bit Operations/Compare To Constant  relop=>  const=10  OutDataTypeStr=boolean
  Compare To Constant2 : simulink/Logic and Bit Operations/Compare To Constant  relop=>  const=10  OutDataTypeStr=boolean
  Constant : Constant  Value=BattBox1_No
  Constant1 : Constant  Value=BattBox2_No
  Constant2 : Constant  Value=BattBox3_No
  Constant6 : Constant  Value=0
  Constant7 : Constant  Value=0
  Constant8 : Constant  Value=0
  Constant9 : Constant  Value=Voltage_NA_UB
  GreaterThan{,1..3} (4 alike) : RelationalOperator  OutDataTypeStr=boolean  RndMeth=Simplest  InputSameDT=off
  GreaterThan{4..7} (4 alike) : RelationalOperator  Operator=<=  OutDataTypeStr=boolean  RndMeth=Simplest  InputSameDT=off
  NOT : Logic  Operator=NOT  AllPortsSameDT=off  OutDataTypeStr=boolean
  NOT1 : Logic  Operator=NOT  AllPortsSameDT=off  OutDataTypeStr=boolean
  NOT2 : Logic  Operator=NOT  AllPortsSameDT=off  OutDataTypeStr=boolean
  Switch{,1..9} (10 alike) : Switch  Criteria=u2 > Threshold  SaturateOnIntegerOverflow=off  InputSameDT=off
  IT_u8BMS_BB_No_MaxVoltage : Outport
  IT_u8BMS_BB_No_MinVoltage : Outport  Port=2
  wires:
  IP_boBMS_Batt3_Availability/1 -> AND9/2
  NOT2/1 -> AND9/1
  IP_boBMS_Batt2_Availability/1 -> AND8/2
  AND7/1 -> AND4/2, Switch4/2
  IP_boBMS_Batt1_Availability/1 -> AND7/2
  AND6/1 -> Switch9/2
  Compare To Constant2/1 -> AND6/1
  AND9/1 -> AND6/2, Switch6/2
  IP_sBMS_VtgInt_BB3/1 -> Switch6/1, Compare To Constant2/1, Switch9/1
  Constant9/1 -> Switch7/3, Switch8/3, Switch9/3
  IP_sBMS_VtgInt_BB2/1 -> Switch5/1, Compare To Constant1/1, Switch8/1
  AND8/1 -> AND5/2, Switch5/2
  Compare To Constant1/1 -> AND5/1
  AND5/1 -> Switch8/2
  AND4/1 -> Switch7/2
  Compare To Constant/1 -> AND4/1
  Switch9/1 -> GreaterThan5/2, GreaterThan7/2
  Switch8/1 -> GreaterThan4/2, GreaterThan6/1, GreaterThan7/1
  Switch7/1 -> GreaterThan4/1, GreaterThan5/1, GreaterThan6/2
  IP_boBMS_SDError_BB1/1 -> NOT/1
  IP_sBMS_VtgInt_BB1/1 -> Compare To Constant/1, Switch7/1, Switch4/1
  IP_boBMS_SDError_BB3/1 -> NOT2/1
  Constant8/1 -> Switch6/3
  IP_boBMS_SDError_BB2/1 -> NOT1/1
  NOT1/1 -> AND8/1
  Constant7/1 -> Switch5/3
  Constant6/1 -> Switch4/3
  NOT/1 -> AND7/1
  GreaterThan7/1 -> AND3/2
  GreaterThan6/1 -> AND3/1
  AND2/1 -> Switch2/2
  Constant/1 -> Switch/1, Switch2/1
  Switch3/1 -> Switch2/3
  Constant1/1 -> Switch1/1, Switch3/1
  Constant2/1 -> Switch1/3, Switch3/3
  AND3/1 -> Switch3/2
  Switch2/1 -> IT_u8BMS_BB_No_MinVoltage/1
  GreaterThan5/1 -> AND2/2
  GreaterThan4/1 -> AND2/1
  Switch/1 -> IT_u8BMS_BB_No_MaxVoltage/1
  AND1/1 -> Switch1/2
  GreaterThan3/1 -> AND1/2
  GreaterThan2/1 -> AND1/1
  Switch1/1 -> Switch/3
  AND/1 -> Switch/2
  GreaterThan1/1 -> AND/2
  GreaterThan/1 -> AND/1
  Switch6/1 -> GreaterThan3/2, GreaterThan1/2
  Switch5/1 -> GreaterThan2/1, GreaterThan/2, GreaterThan3/1
  Switch4/1 -> GreaterThan1/1, GreaterThan2/2, GreaterThan/1

== system ChiefMaster_TTC580/ChiefMaster/Input Translation/Battery Signals/Subsystem/Subsystem ==
  <IP_sBatt1_Ubatt_Databus> : Inport
  <IP_LB_BMS_Pack_V_Cells_DataBus> : Inport  Port=2
  Bus Selector2 : BusSelector  OutputSignals=sData
  Bus Selector5 : BusSelector  OutputSignals=sData
  Constant : Constant  Value=0  OutDataTypeStr=single
  Multiport Switch : MultiPortSwitch  DataPortForDefault=Additional data port  DiagnosticForDefault=None  SaturateOnIntegerOverflow=off  InputSameDT=off
  IP_sBMS_VtgInt_BB1 : Outport
  wires:
  Bus Selector2/1 -> Multiport Switch/2  "<sData>"
  [Select_Battery1] -> Multiport Switch/1
  Multiport Switch/1 -> IP_sBMS_VtgInt_BB1/1  "IP_sBMS_VtgInt_BB1"
  <IP_LB_BMS_Pack_V_Cells_DataBus>/1 -> Bus Selector5/1
  Constant/1 -> Multiport Switch/5, Multiport Switch/4
  Bus Selector5/1 -> Multiport Switch/3  "<sData>"
  <IP_sBatt1_Ubatt_Databus>/1 -> Bus Selector2/1

== system ChiefMaster_TTC580/ChiefMaster/Input Translation/Battery Signals/Subsystem/Subsystem1 ==
  <IP_sBatt2_Ubatt_Databus> : Inport
  <IP_LB_BMS_Pack_V_Cells_DataBus> : Inport  Port=2
  Bus Selector2 : BusSelector  OutputSignals=sData
  Bus Selector5 : BusSelector  OutputSignals=sData
  Constant : Constant  Value=0  OutDataTypeStr=single
  Multiport Switch : MultiPortSwitch  DataPortForDefault=Additional data port  DiagnosticForDefault=None  SaturateOnIntegerOverflow=off  InputSameDT=off
  IP_sBMS_VtgInt_BB2 : Outport
  wires:
  <IP_sBatt2_Ubatt_Databus>/1 -> Bus Selector2/1
  Bus Selector5/1 -> Multiport Switch/3  "<sData>"
  Constant/1 -> Multiport Switch/4, Multiport Switch/5
  <IP_LB_BMS_Pack_V_Cells_DataBus>/1 -> Bus Selector5/1
  Multiport Switch/1 -> IP_sBMS_VtgInt_BB2/1  "IP_sBMS_VtgInt_BB2"
  [Select_Battery2] -> Multiport Switch/1
  Bus Selector2/1 -> Multiport Switch/2  "<sData>"

== system ChiefMaster_TTC580/ChiefMaster/Input Translation/Battery Signals/Subsystem/Subsystem2 ==
  <IP_sBatt3_Ubatt_Databus> : Inport
  <IP_LB_BMS_Pack_V_Cells_DataBus> : Inport  Port=2
  Bus Selector2 : BusSelector  OutputSignals=sData
  Bus Selector5 : BusSelector  OutputSignals=sData
  Constant : Constant  Value=0  OutDataTypeStr=single
  Multiport Switch : MultiPortSwitch  DataPortForDefault=Additional data port  DiagnosticForDefault=None  SaturateOnIntegerOverflow=off  InputSameDT=off
  IP_sBMS_VtgInt_BB3 : Outport
  wires:
  Bus Selector2/1 -> Multiport Switch/2  "<sData>"
  [Select_Battery3] -> Multiport Switch/1
  Multiport Switch/1 -> IP_sBMS_VtgInt_BB3/1  "IP_sBMS_VtgInt_BB3"
  <IP_LB_BMS_Pack_V_Cells_DataBus>/1 -> Bus Selector5/1
  Constant/1 -> Multiport Switch/5, Multiport Switch/4
  Bus Selector5/1 -> Multiport Switch/3  "<sData>"
  <IP_sBatt3_Ubatt_Databus>/1 -> Bus Selector2/1

== system ChiefMaster_TTC580/ChiefMaster/Input Translation/Battery Signals/Subsystem1/Subsystem ==
  <IP_boBatt1_SDERR_activ> : Inport
  <IP_LB_Batt1_Status01_DataBus> : Inport  Port=2
  Bus Selector : BusSelector  OutputSignals=IP_u8LB_BMS_Status
  Compare To Constant : simulink/Logic and Bit Operations/Compare To Constant  relop===  const=4  OutDataTypeStr=boolean
  Constant : Constant  Value=0  OutDataTypeStr=boolean
  Multiport Switch : MultiPortSwitch  DataPortForDefault=Additional data port  DiagnosticForDefault=Warning  SaturateOnIntegerOverflow=off  InputSameDT=off
  IP_boBMS_SDError_BB1 : Outport
  wires:
  Compare To Constant/1 -> Multiport Switch/3
  <IP_LB_Batt1_Status01_DataBus>/1 -> Bus Selector/1
  <IP_boBatt1_SDERR_activ>/1 -> Multiport Switch/2
  Constant/1 -> Multiport Switch/5, Multiport Switch/4
  Bus Selector/1 -> Compare To Constant/1  "<IP_u8LB_BMS_Status>"
  [Select_Battery1] -> Multiport Switch/1
  Multiport Switch/1 -> IP_boBMS_SDError_BB1/1  "IP_boBMS_SDError_BB1"

== system ChiefMaster_TTC580/ChiefMaster/Input Translation/Battery Signals/Subsystem1/Subsystem1 ==
  <IP_boBatt2_SDERR_activ> : Inport
  <IP_LB_Batt2_Status01_DataBus> : Inport  Port=2
  Bus Selector : BusSelector  OutputSignals=IP_u8LB_BMS_Status
  Compare To Constant : simulink/Logic and Bit Operations/Compare To Constant  relop===  const=4  OutDataTypeStr=boolean
  Constant : Constant  Value=0  OutDataTypeStr=boolean
  Multiport Switch : MultiPortSwitch  DataPortForDefault=Additional data port  DiagnosticForDefault=Warning  SaturateOnIntegerOverflow=off  InputSameDT=off
  IP_boBMS_SDError_BB2 : Outport
  wires:
  Compare To Constant/1 -> Multiport Switch/3
  Constant/1 -> Multiport Switch/5, Multiport Switch/4
  Bus Selector/1 -> Compare To Constant/1  "<IP_u8LB_BMS_Status>"
  Multiport Switch/1 -> IP_boBMS_SDError_BB2/1  "IP_boBMS_SDError_BB2"
  <IP_boBatt2_SDERR_activ>/1 -> Multiport Switch/2
  [Select_Battery2] -> Multiport Switch/1
  <IP_LB_Batt2_Status01_DataBus>/1 -> Bus Selector/1

== system ChiefMaster_TTC580/ChiefMaster/Input Translation/Battery Signals/Subsystem1/Subsystem2 ==
  <IP_boBatt3_SDERR_activ> : Inport
  <IP_LB_Batt2_Status01_DataBus> : Inport  Port=2
  Bus Selector : BusSelector  OutputSignals=IP_u8LB_BMS_Status
  Compare To Constant : simulink/Logic and Bit Operations/Compare To Constant  relop===  const=4  OutDataTypeStr=boolean
  Constant : Constant  Value=0  OutDataTypeStr=boolean
  Multiport Switch : MultiPortSwitch  DataPortForDefault=Additional data port  DiagnosticForDefault=Warning  SaturateOnIntegerOverflow=off  InputSameDT=off
  IP_boBMS_SDError_BB3 : Outport
  wires:
  <IP_LB_Batt2_Status01_DataBus>/1 -> Bus Selector/1
  [Select_Battery3] -> Multiport Switch/1
  <IP_boBatt3_SDERR_activ>/1 -> Multiport Switch/2
  Multiport Switch/1 -> IP_boBMS_SDError_BB3/1  "IP_boBMS_SDError_BB3"
  Bus Selector/1 -> Compare To Constant/1  "<IP_u8LB_BMS_Status>"
  Constant/1 -> Multiport Switch/4, Multiport Switch/5
  Compare To Constant/1 -> Multiport Switch/3

== system ChiefMaster_TTC580/ChiefMaster/Input Translation/Battery Signals/Subsystem10/Subsystem1 ==
  <IP_boBMS_IMD_Active_BB2> : Inport
  IMD_Req_Databus : Inport  Port=2
  Bus Selector : BusSelector  OutputSignals=FL_IMD_Control_Databus.FL_boREQ_IMD_ON_BB2
  Constant : Constant  Value=0  OutDataTypeStr=boolean
  Delay : Delay  DelayLength=3
  Multiport Switch : MultiPortSwitch  DataPortForDefault=Additional data port  DiagnosticForDefault=Warning  SaturateOnIntegerOverflow=off  InputSameDT=off
  IP_boBMS_IMD_Active_BB2 : Outport  OutDataTypeStr=boolean
  wires:
  Constant/1 -> Multiport Switch/5, Multiport Switch/4
  [Select_Battery2] -> Multiport Switch/1
  <IP_boBMS_IMD_Active_BB2>/1 -> Multiport Switch/2
  Multiport Switch/1 -> IP_boBMS_IMD_Active_BB2/1  "IP_boBMS_IMD_Active_BB2"
  Delay/1 -> Multiport Switch/3
  Bus Selector/1 -> Delay/1  "<FL_boREQ_IMD_ON_BB2>"
  IMD_Req_Databus/1 -> Bus Selector/1

== system ChiefMaster_TTC580/ChiefMaster/Input Translation/Battery Signals/Subsystem10/Subsystem2 ==
  <IP_boBMS_IMD_Active_BB3> : Inport
  IMD_Req_Databus : Inport  Port=2
  Bus Selector : BusSelector  OutputSignals=FL_IMD_Control_Databus.FL_boREQ_IMD_ON_BB3
  Constant : Constant  Value=0  OutDataTypeStr=boolean
  Delay : Delay  DelayLength=3
  Multiport Switch : MultiPortSwitch  DataPortForDefault=Additional data port  DiagnosticForDefault=Warning  SaturateOnIntegerOverflow=off  InputSameDT=off
  IP_boBMS_IMD_Active_BB3 : Outport  OutDataTypeStr=boolean
  wires:
  Multiport Switch/1 -> IP_boBMS_IMD_Active_BB3/1  "IP_boBMS_IMD_Active_BB3"
  <IP_boBMS_IMD_Active_BB3>/1 -> Multiport Switch/2
  [Select_Battery3] -> Multiport Switch/1
  Constant/1 -> Multiport Switch/4, Multiport Switch/5
  IMD_Req_Databus/1 -> Bus Selector/1
  Bus Selector/1 -> Delay/1  "<FL_boREQ_IMD_ON_BB3>"
  Delay/1 -> Multiport Switch/3
